simulink model "rt_uebung2"  (Simulink 8.1)
settings: Solver=ode45  StartTime=0.0  StopTime=10.0  RelTol=1e-3
settings Model: Creator=mainster  LastModifiedBy=mainster

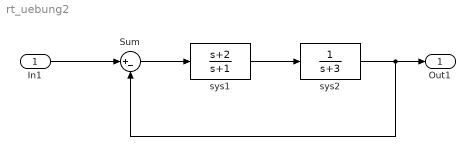
== system rt_uebung2 ==
  In1 : Inport
  Sum : Sum  Inputs=|+-
  sys1 : TransferFcn  Numerator=[1 2]  Denominator=[1 1]
  sys2 : TransferFcn  Denominator=[1 3]
  Out1 : Outport
  wires:
  In1/1 -> Sum/1
  Sum/1 -> sys1/1
  sys1/1 -> sys2/1
  sys2/1 -> Sum/2, Out1/1
